simulink model "mconversionToFile"  (Simulink 6.0)
settings: Solver=ode45  StartTime=0.0  StopTime=10.0  RelTol=1e-3
settings Model: Creator=awarlock  LastModifiedBy=awarlock  ExtModeAutoUpdateStatusClock=off

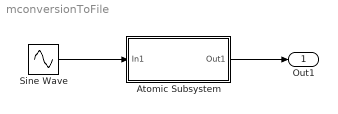
== system mconversionToFile ==
  Atomic Subsystem : Subsystem  TreatAsAtomicUnit=on
  Sine Wave : Sin  SampleTime=0.1
  Out1 : Outport
  wires:
  Sine Wave/1 -> Atomic Subsystem/1(In1)
  Atomic Subsystem/1(Out1) -> Out1/1

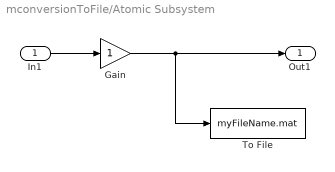
== system mconversionToFile/Atomic Subsystem ==
  In1 : Inport  Port=1  LatchInput=off
  Gain : Gain
  To File : ToFile  Filename=myFileName.mat
  Out1 : Outport
  wires:
  In1/1 -> Gain/1
  Gain/1 -> Out1/1, To File/1
